simulink model "state_feedback_2wbr"  (R2017b)
settings: Solver=VariableStepAuto  StartTime=0.0  StopTime=10.0  RelTol=1e-3
settings Model: Creator=Iman  LastModifiedBy=Iman

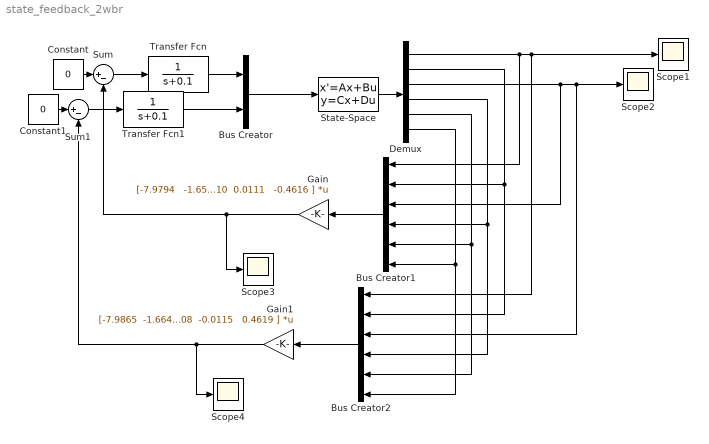
== system state_feedback_2wbr ==
  Bus Creator : BusCreator  Inputs=2
  Bus Creator1 : BusCreator  Inputs=6
  Bus Creator2 : BusCreator  Inputs=6
  Constant : Constant  Value=0
  Constant1 : Constant  Value=0
  Demux : Demux  Outputs=6
  Gain : Gain  Gain=|  Multiplication=Matrix(K*u)
      | [-7.9794   -1.6598   -1.0692   -0.1310  0.0111   -0.4616
      | ]
  Gain1 : Gain  Gain=|  Multiplication=Matrix(K*u)
      | [-7.9865  -1.6642  -1.0686   -0.1308  -0.0115   0.4619
      | ]
  Scope{1..4} (4 alike) : Scope
  State-Space : StateSpace  A=[0 1 0 0 0 0;0 -1690 -23 68 0 0;0 0 0 1 0 0;0 21481 370 -859 0 0;0 0 0 0 0 1;0 0 0 0 0 -610]  B=[0 0;104.5 104.5;0 0;-1373.8 -1373.8;0 0;650.2 -650.2]  C=[1 0 0 0 0 0;0 1 0 0 0 0;0 0 1 0 0 0;0 0 0 1 0 0;0 0 0 0 1 0;0 0 0 0 0 1]  D=[0 0;0 0;0 0;0 0;0 0;0 0]  InitialCondition=[0 0 0.15 0 0 0]
  Sum : Sum  Inputs=|+-
  Sum1 : Sum  Inputs=|+-
  Transfer Fcn : TransferFcn  Denominator=[1 0.1]
  Transfer Fcn1 : TransferFcn  Denominator=[1 0.1]
  wires:
  Constant/1 -> Sum/1
  State-Space/1 -> Demux/1
  Bus Creator/1 -> State-Space/1
  Sum/1 -> Transfer Fcn/1
  Constant1/1 -> Sum1/1
  Sum1/1 -> Transfer Fcn1/1
  Bus Creator1/1 -> Gain/1
  Demux/2 -> Bus Creator2/2, Bus Creator1/2
  Demux/3 -> Bus Creator1/3, Bus Creator2/3, Scope2/1
  Demux/4 -> Bus Creator2/4, Bus Creator1/4
  Demux/1 -> Bus Creator1/1, Bus Creator2/1, Scope1/1
  Demux/6 -> Bus Creator2/6, Bus Creator1/6
  Demux/5 -> Bus Creator2/5, Bus Creator1/5
  Bus Creator2/1 -> Gain1/1
  Gain/1 -> Scope3/1, Sum/2
  Gain1/1 -> Scope4/1, Sum1/2
  Transfer Fcn/1 -> Bus Creator/1
  Transfer Fcn1/1 -> Bus Creator/2
